simulink model "HILModelFull"  (Simulink 6.6)
settings: Solver=ode4  StartTime=0.0  StopTime=inf  FixedStep=SampleT  RelTol=1e-3
InitFcn:
  | clc
  | Taxi_Var_new
  | failures
  | insInit
  | piccolo_init
values from neighbouring files (symbols this model uses):
  A1 = 0    [Taxi_Var.m]
  Apolar = 0.0899    [Taxi_Var.m]
  CD0 = 0.0219    [Taxi_Var.m]
  chord = S/span    (= 0.384036716878)    [Taxi_Var.m]
  CL0 = 0.1857    [Taxi_Var.m]
  CLa = 4.6206    [Taxi_Var.m]
  CLa_dot = 1.93    [Taxi_Var.m]
  Clb = -0.0043    [Taxi_Var.m]
  ClDa = 0.1695    [Taxi_Var.m]
  CLDe = 0.4032    [Taxi_Var.m]
  CLDf = 0.047    [Taxi_Var.m]
  ClDr = 0.0003    [Taxi_Var.m]
  Clp = -0.4425    [Taxi_Var.m]
  CLq = 8.7465    [Taxi_Var.m]
  Clr = 0.0675    [Taxi_Var.m]
  Cm0 = -0.0902    [Taxi_Var.m]
  Cma = -1.3995    [Taxi_Var.m]
  CmDe = -0.9493    [Taxi_Var.m]
  CmDf = -.021    (= -0.021)    [Taxi_Var.m]
  Cmq = -10.8760    (= -10.876)    [Taxi_Var.m]
  Cnb = 0.0281    [Taxi_Var.m]
  CnDa = -0.0031    [Taxi_Var.m]
  CnDr = -0.0882    [Taxi_Var.m]
  Cnp = -0.0695    [Taxi_Var.m]
  Cnr = -0.1045    [Taxi_Var.m]
  CYb = -0.1999    [Taxi_Var.m]
  CYDr = 0.0192    [Taxi_Var.m]
  damax = 25*deg2rad    (= 0.436332312999)    [Taxi_Var.m]
  damin = -25*deg2rad    (= -0.436332312999)    [Taxi_Var.m]
  datrim = 0*deg2rad    (= 0)    [Taxi_Var.m]
  demax = 15*deg2rad    (= 0.261799387799)    [Taxi_Var.m]
  demin = -15*deg2rad    (= -0.261799387799)    [Taxi_Var.m]
  detrim = -2.4137*deg2rad    (= -0.0421270121554)    [Taxi_Var.m]
  dfland = 30*deg2rad    (= 0.523598775598)    [Taxi_Var.m]
  dfmax = 30*deg2rad    (= 0.523598775598)    [Taxi_Var.m]
  dfmin = 0*deg2rad    (= 0)    [Taxi_Var.m]
  drmax = 25*deg2rad    (= 0.436332312999)    [Taxi_Var.m]
  drmin = -25*deg2rad    (= -0.436332312999)    [Taxi_Var.m]
  drtrim = 0*deg2rad    (= 0)    [Taxi_Var.m]
  dtmax = 1    [Taxi_Var.m]
  dtmin = 0    [Taxi_Var.m]
  dttrim = 0.0725    [Taxi_Var.m]
  Euler_0 = [0; 0; 45]'*pi/180    [Taxi_Var.m]    (also in hilInit.m = [0; 0; 0*pi/180]')
  HIL_K = 3    [hilInit.m]    (also in insInit.m)
  ISA_g = 9.815    [Taxi_Var.m]
  ISA_hmax = 2000    [Taxi_Var.m]
  ISA_lapse = .0065    (= 0.0065)    [Taxi_Var.m]
  ISA_P0 = 101325    [Taxi_Var.m]
  ISA_R = 287    [Taxi_Var.m]
  ISA_rho0 = 1.225    [Taxi_Var.m]
  ISA_T0 = 289    [Taxi_Var.m]
  Ixx = 3.689084    [Taxi_Var.m]
  Iyy = 7.43789    [Taxi_Var.m]
  Izz = 10.22202    [Taxi_Var.m]
  mass = 22.5    [Taxi_Var.m]
  MinThK = 0.075    [Taxi_Var.m]
  Pos_0 = [0; 0; 1000]'    [Taxi_Var.m]    (also in hilInit.m = [500; 750; 350]')
  PQR_0 = [0; 0; 0]'    [Taxi_Var.m]
  span = 2.3368    [Taxi_Var.m]
  TFact = 0.4    [Taxi_Var.m]
  ThK = 2.18    [Taxi_Var.m]
  Vb_0 = [35; 0; 0]'    [Taxi_Var.m]
undefined symbols (not defined in the file or in its folder): clock, Earth, IdxCmdOrbitRadius, IdxCmdOrbitSense, IdxCmdWp1Alt, IdxCmdWp1Lat, IdxCmdWp1Lon, IdxCmdWp2Alt, IdxCmdWp2Lat, IdxCmdWp2Lon, IdxEstimReserved1, IdxEstimWEast, IdxEstimWNorth, IdxGainsAltD, IdxGainsAltI, IdxGainsAltP, IdxGainsPdynD, IdxGainsPdynI, IdxGainsPdynP, IdxGainsPitchD, IdxGainsPitchI, IdxGainsPitchP, IdxGainsRollD, IdxGainsRollI, IdxGainsRollP, IdxGainsSlopeElevatorD, IdxGainsSlopeElevatorP, IdxGainsTrackConv, IdxGainsTrackD, IdxGainsTrackI, IdxGainsTrackP, IdxGainsTurnD, IdxGainsTurnI, IdxGainsTurnP, IdxGainsYawD, IdxGainsYawI, IdxGainsYawP, IdxLimitsAileronMax, IdxLimitsAileronMin, IdxLimitsBankMax, IdxLimitsBankMin, IdxLimitsElevatorMax, IdxLimitsElevatorMin, IdxLimitsFlapMax, IdxLimitsFlapMin, IdxLimitsPdynMax, IdxLimitsPdynMin, IdxLimitsRudderMax, IdxLimitsRudderMin, IdxLimitsThrottleMax, IdxLimitsThrottleMin, IdxSensorsAlt, IdxSensorsLat, IdxSensorsLon, IdxSensorsVDown, IdxSensorsVEast, IdxSensorsVNorth, IdxStatesGlobal, IdxStatesManual, IdxStatesMode ... (+3)
libraries: piccolo_library x60, simulink x33, xpclib x8, aerolibasang x5, aerolibconvert2 x5, aerolibtransform2 x2, aerolibnav x2, aerolibatmos2 x1, dspmtrx3 x1
(part 1 of 4)
CloseFcn:
  | rtwprivate ssgencode ModelCloseRequest AttitudeComplementary
settings Model: Creator=ASL_Lab  LastModifiedBy=UavlabUser
settings DebuggingCC: AlgebraicLoopMsg=error  MultiTaskDSMMsg=warning  MultiTaskCondExecSysMsg=none  StrictBusMsg=None
settings HardwareCC: TargetHWDeviceType=32-bit Generic
settings RTWCC: IncludeERTFirstTime=on

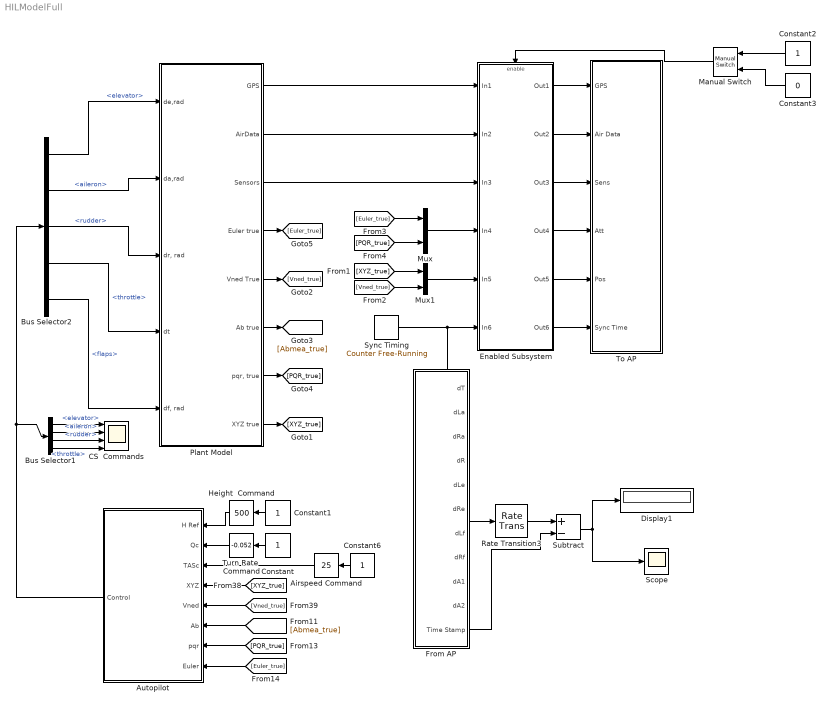
== system HILModelFull ==
  Airspeed Command : simulink/Math Operations/Slider Gain  Orientation=left  SystemSampleTime=-1  low=15  gain=25  high=50
  Autopilot : Subsystem  Orientation=left
  Bus Selector1 : BusSelector  OutputSignals=elevator,aileron,rudder,throttle
  Bus Selector2 : BusSelector  OutputSignals=elevator,aileron,rudder,throttle,flaps
  CS  Commands : Scope  NumInputPorts=4
      settings: TimeRange=44  YMin=0.0142~-2.5e-018~-1e-017~0.665  YMax=0.014425~2e-018~1e-017~0.735  SaveName=ScopeData19
  Constant{,1..2,6} (4 alike) : Constant  Orientation=left
  Constant3 : Constant  Orientation=left  Value=0
  Display1 : Display
  Enabled Subsystem : Subsystem  TreatAsAtomicUnit=on
  From AP : Subsystem
  Height  Command : simulink/Math Operations/Slider Gain  Orientation=left  SystemSampleTime=-1  low=150  gain=500  high=1500
  Manual Switch : simulink/Signal Routing/Manual Switch  Orientation=left  SystemSampleTime=-1  sw=1  action=0  varsize=off
  Mux : Mux  Inputs=2
  Mux1 : Mux  Inputs=2
  Plant Model : Subsystem
  Rate Transition3 : RateTransition  OutPortSampleTime=SampleT
  Scope : Scope
      settings: SaveName=ScopeData2
  Subtract : Sum  Inputs=+-  OutScaling=2^-10
  Sync Timing : simulink/Sources/Counter Free-Running  SystemSampleTime=-1  NumBits=16  tsamp=SampleT*HIL_K
  To AP : Subsystem
  Turn Rate  Command : simulink/Math Operations/Slider Gain  Orientation=left  SystemSampleTime=-1  low=-0.2  gain=-0.052  high=0.2
  wires:
  [XYZ_true] -> Autopilot/4(XYZ)
  [Vned_true] -> Autopilot/5(Vned)
  [Abmea_true] -> Autopilot/6(Ab)
  [PQR_true] -> Autopilot/7(pqr)
  [Euler_true] -> Autopilot/8(Euler)
  Autopilot/1(Control) -> Bus Selector2/1, Bus Selector1/1
  Bus Selector2/1 -> Plant Model/1(de,rad)  "<elevator>"
  Bus Selector2/2 -> Plant Model/2(da,rad)  "<aileron>"
  Bus Selector2/3 -> Plant Model/3("dr, rad")  "<rudder>"
  Bus Selector2/4 -> Plant Model/4(dt)  "<throttle>"
  Bus Selector2/5 -> Plant Model/5("df, rad")  "<flaps>"
  Bus Selector1/1 -> CS  Commands/1  "<elevator>"
  Bus Selector1/2 -> CS  Commands/2  "<aileron>"
  Bus Selector1/3 -> CS  Commands/3  "<rudder>"
  Bus Selector1/4 -> CS  Commands/4  "<throttle>"
  Constant/1 -> Turn Rate  Command/1
  Turn Rate  Command/1 -> Autopilot/2(Qc)
  Constant1/1 -> Height  Command/1
  Height  Command/1 -> Autopilot/1(H Ref)
  Constant6/1 -> Airspeed Command/1
  Airspeed Command/1 -> Autopilot/3(TASc)
  Plant Model/8(XYZ true) -> [XYZ_true]
  Plant Model/5(Vned True) -> [Vned_true]
  Plant Model/6(Ab true) -> [Abmea_true]
  Plant Model/7("pqr, true") -> [PQR_true]
  Plant Model/4(Euler true) -> [Euler_true]
  [PQR_true] -> Mux/2
  [XYZ_true] -> Mux1/1
  [Vned_true] -> Mux1/2
  [Euler_true] -> Mux/1
  Enabled Subsystem/1(Out1) -> To AP/1(GPS)
  Enabled Subsystem/2(Out2) -> To AP/2(Air Data)
  Enabled Subsystem/3(Out3) -> To AP/3(Sens)
  Enabled Subsystem/4(Out4) -> To AP/4(Att)
  Enabled Subsystem/5(Out5) -> To AP/5(Pos)
  Enabled Subsystem/6(Out6) -> To AP/6(Sync Time)
  Plant Model/1(GPS) -> Enabled Subsystem/1(In1)
  Plant Model/2(AirData) -> Enabled Subsystem/2(In2)
  Plant Model/3(Sensors) -> Enabled Subsystem/3(In3)
  Mux/1 -> Enabled Subsystem/4(In4)
  Mux1/1 -> Enabled Subsystem/5(In5)
  Sync Timing/1 -> Enabled Subsystem/6(In6), Rate Transition3/1
  Manual Switch/1 -> Enabled Subsystem/Enable
  Constant2/1 -> Manual Switch/1
  Constant3/1 -> Manual Switch/2
  From AP/11(Time Stamp) -> Subtract/2
  Subtract/1 -> Display1/1, Scope/1
  Rate Transition3/1 -> Subtract/1

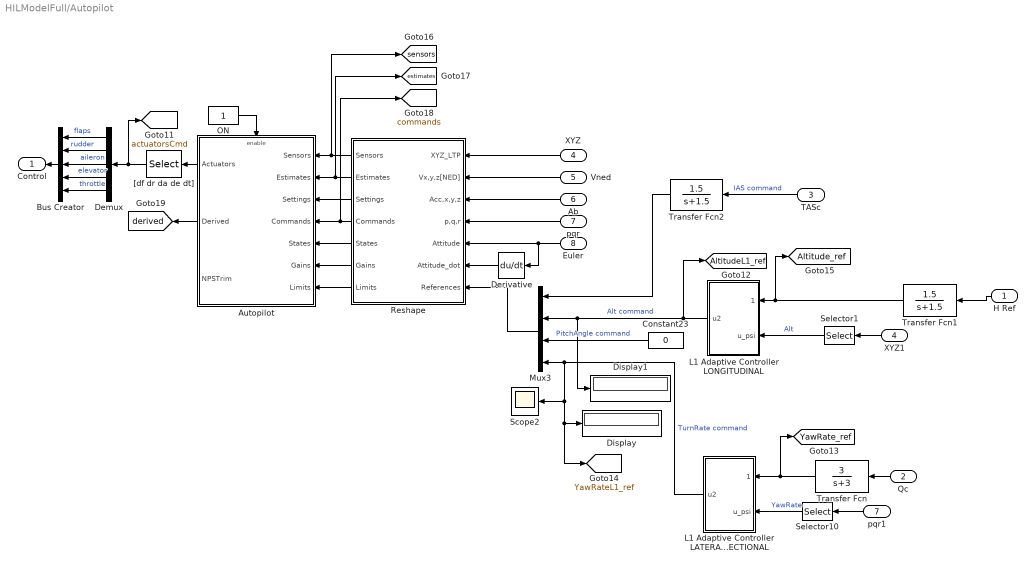
== system HILModelFull/Autopilot ==
  H Ref : Inport  Orientation=left
  Qc : Inport  Orientation=left  Port=2
  TASc : Inport  Orientation=left  Port=3
  XYZ : Inport  Orientation=left  Port=4
  Vned : Inport  Orientation=left  Port=5
  Ab : Inport  Orientation=left  Port=6
  pqr : Inport  Orientation=left  Port=7
  Euler : Inport  Orientation=left  Port=8
  Autopilot : Subsystem  Orientation=left
  Bus Creator : BusCreator  Orientation=left  Inputs=5
  Constant23 : Constant  Orientation=left  Value=0
  Demux : Demux  Orientation=left  Outputs=5
  Derivative : Derivative  Orientation=left
  Display : Display
  Display1 : Display
  L1 Adaptive Controller LATERAL-DIRECTIONAL : Subsystem  Orientation=left  mask{gamma=-2000, m=4, omega=2, Pbound=.1, L1ONOFF=0}
      mask prompts: gamma "L1 gain"; m "state predictor (m)"; omega "low-pass filter (omega)"; Pbound "projection bounds"; L1ONOFF "L1 switch"
  L1 Adaptive Controller LONGITUDINAL : Subsystem  Orientation=left  mask{gamma=-1, m=4, omega=1, Pbound=50, L1ONOFF=0}
      mask prompts: gamma "L1 gain"; m "state predictor (m)"; omega "low-pass filter (omega)"; Pbound "projection bounds"; L1ONOFF "L1 switch"
  Mux3 : Mux  Orientation=left
  ON : Constant
  Reshape : Subsystem  Orientation=left
  Scope2 : Scope
      settings: YMin=-1  YMax=1  SaveName=ScopeData29
  Selector1 : Selector  Orientation=left  IndexOptions=Index vector (dialog)  Indices=3  OutputSizes=1  InputPortWidth=3
  Selector10 : Selector  Orientation=left  IndexOptions=Index vector (dialog)  Indices=3  OutputSizes=1  InputPortWidth=3
  Transfer Fcn : TransferFcn  Orientation=left  Numerator=[3]  Denominator=[1 3]
  Transfer Fcn1 : TransferFcn  Orientation=left  Numerator=[1.5]  Denominator=[1 1.5]
  Transfer Fcn2 : TransferFcn  Orientation=left  Numerator=[1.5]  Denominator=[1 1.5]
  XYZ1 : InportShadow  Orientation=left  Port=4  LatchByCopyingInsideSignal=off
  "[df dr da de dt]" : Selector  Orientation=left  IndexOptions=Index vector (dialog)  Indices=[10 6 2 4 8]  OutputSizes=[(-2)]  InputPortWidth=12
  pqr1 : InportShadow  Orientation=left  Port=7  LatchByCopyingInsideSignal=off
  Control : Outport  Orientation=left
  tag scope: AltitudeL1_ref=global, Altitude_ref=global, YawRateL1_ref=global, YawRate_ref=global, actuatorsCmd=global, commands=global, derived=global, estimates=global, sensors=global
  wires:
  XYZ/1 -> Reshape/1(XYZ_LTP)
  Vned/1 -> Reshape/2(Vx,y,z[NED])
  Ab/1 -> Reshape/3(Acc,x,y,z)
  pqr/1 -> Reshape/4(p,q,r)
  Reshape/1(Sensors) -> Autopilot/1(Sensors), [sensors]
  Reshape/2(Estimates) -> Autopilot/2(Estimates), [estimates]
  Reshape/3(Settings) -> Autopilot/3(Settings)
  Reshape/4(Commands) -> Autopilot/4(Commands), [commands]
  Reshape/5(States) -> Autopilot/5(States)
  Reshape/6(Gains) -> Autopilot/6(Gains)
  Reshape/7(Limits) -> Autopilot/7(Limits)
  ON/1 -> Autopilot/Enable
  Autopilot/1(Actuators) -> "[df dr da de dt]"/1
  "[df dr da de dt]"/1 -> Demux/1, [actuatorsCmd]
  Euler/1 -> Reshape/5(Attitude), Derivative/1
  Autopilot/2(Derived) -> [derived]
  TASc/1 -> Transfer Fcn2/1  "IAS command"
  L1 Adaptive Controller LONGITUDINAL/1(u2) -> [AltitudeL1_ref], Mux3/2, Display1/1  "Alt command"
  Constant23/1 -> Mux3/3  "PitchAngle command"
  L1 Adaptive Controller LATERAL-DIRECTIONAL/1(u2) -> Mux3/4, Display/1, [YawRateL1_ref], Scope2/1  "TurnRate command"
  Mux3/1 -> Reshape/7(References)
  Qc/1 -> Transfer Fcn/1
  pqr1/1 -> Selector10/1
  Selector10/1 -> L1 Adaptive Controller LATERAL-DIRECTIONAL/2(u_psi)  "YawRate"
  H Ref/1 -> Transfer Fcn1/1
  XYZ1/1 -> Selector1/1
  Selector1/1 -> L1 Adaptive Controller LONGITUDINAL/2(u_psi)  "Alt"
  Demux/1 -> Bus Creator/1  "flaps"
  Demux/2 -> Bus Creator/2  "rudder"
  Demux/3 -> Bus Creator/3  "aileron"
  Demux/4 -> Bus Creator/4  "elevator"
  Demux/5 -> Bus Creator/5  "throttle"
  Bus Creator/1 -> Control/1
  Transfer Fcn/1 -> L1 Adaptive Controller LATERAL-DIRECTIONAL/1(u_psi_c), [YawRate_ref]
  Transfer Fcn1/1 -> L1 Adaptive Controller LONGITUDINAL/1(u_psi_c), [Altitude_ref]
  Transfer Fcn2/1 -> Mux3/1
  Derivative/1 -> Reshape/6(Attitude_dot)

== system HILModelFull/Enabled Subsystem ==
  In1 : Inport
  In2 : Inport  Port=2
  In3 : Inport  Port=3
  In4 : Inport  Port=4
  In5 : Inport  Port=5
  In6 : Inport  Port=6
  Enable : EnablePort
  Out1 : Outport
  Out2 : Outport  Port=2
  Out3 : Outport  Port=3
  Out4 : Outport  Port=4
  Out5 : Outport  Port=5
  Out6 : Outport  Port=6
  wires:
  In1/1 -> Out1/1
  In2/1 -> Out2/1
  In3/1 -> Out3/1
  In4/1 -> Out4/1
  In5/1 -> Out5/1
  In6/1 -> Out6/1

== system HILModelFull/From AP ==
  Bus Creator : BusCreator  Inputs=11
  Bus Selector : BusSelector  OutputSignals=dt,dla,dra,dr,dle,dre,dlf,drf,da1,da2,timeStamp
  Data Type Conversion{1..11} (11 alike) : DataTypeConversion  OutDataTypeMode=double
  Receive : xpclib/UDP/Receive  ipAddress=0.0.0.0  ipPort=5678  width=22  sampletime=SampleT
  Terminator : Terminator
  Unpack1 : xpclib/UDP/Unpack  dimensions={1,1,1,1,1,1,1,1,1,1,1}  datatypes={'uint16','uint16','uint16','uint16', 'uint16', 'uint16','uint16', 'uint16','uint16', 'uint16','uint16'}  byteAlign=1
  dT : Outport
  dLa : Outport  Port=2
  dRa : Outport  Port=3
  dR : Outport  Port=4
  dLe : Outport  Port=5
  dRe : Outport  Port=6
  dLf : Outport  Port=7
  dRf : Outport  Port=8
  dA1 : Outport  Port=9
  dA2 : Outport  Port=10
  Time Stamp : Outport  Port=11
  wires:
  Receive/1 -> Unpack1/1
  Receive/2 -> Terminator/1
  Bus Creator/1 -> Bus Selector/1
  Data Type Conversion1/1 -> dT/1
  Data Type Conversion2/1 -> dLa/1
  Data Type Conversion3/1 -> dRa/1
  Data Type Conversion4/1 -> dR/1
  Data Type Conversion5/1 -> dLe/1
  Data Type Conversion6/1 -> dRe/1
  Data Type Conversion7/1 -> dLf/1
  Data Type Conversion8/1 -> dRf/1
  Data Type Conversion9/1 -> dA1/1
  Data Type Conversion10/1 -> dA2/1
  Unpack1/1 -> Bus Creator/1  "dt"
  Unpack1/3 -> Bus Creator/3  "dra"
  Unpack1/5 -> Bus Creator/5  "dle"
  Unpack1/7 -> Bus Creator/7  "dlf"
  Unpack1/9 -> Bus Creator/9  "da1"
  Unpack1/11 -> Bus Creator/11  "timeStamp"
  Data Type Conversion11/1 -> Time Stamp/1
  Bus Selector/1 -> Data Type Conversion1/1  "<dt>"
  Bus Selector/2 -> Data Type Conversion2/1  "<dla>"
  Bus Selector/3 -> Data Type Conversion3/1  "<dra>"
  Bus Selector/4 -> Data Type Conversion4/1  "<dr>"
  Bus Selector/5 -> Data Type Conversion5/1  "<dle>"
  Bus Selector/6 -> Data Type Conversion6/1  "<dre>"
  Bus Selector/7 -> Data Type Conversion7/1  "<dlf>"
  Bus Selector/8 -> Data Type Conversion8/1  "<drf>"
  Bus Selector/9 -> Data Type Conversion9/1  "<da1>"
  Bus Selector/10 -> Data Type Conversion10/1  "<da2>"
  Bus Selector/11 -> Data Type Conversion11/1  "<timeStamp>"
  Unpack1/2 -> Bus Creator/2  "dla"
  Unpack1/4 -> Bus Creator/4  "dr"
  Unpack1/6 -> Bus Creator/6  "dre"
  Unpack1/8 -> Bus Creator/8  "drf"
  Unpack1/10 -> Bus Creator/10  "da2"

== system HILModelFull/Plant Model ==
  de,rad : Inport
  da,rad : Inport  Port=2
  "dr, rad" : Inport  Port=3
  dt : Inport  Port=4
  "df, rad" : Inport  Port=5
  Angle Conversion{,1..3} (4 alike) : aerolibconvert2/Angle Conversion  SystemSampleTime=-1  IU=rad  OU=deg
  Constant : Constant  Value=18  SampleTime=SampleT
  Constant1 : Constant  SampleTime=SampleT
  Constant2 : Constant  Value=7  SampleTime=SampleT
  Constant3 : Constant  SampleTime=SampleT
  Generic Sensor : Subsystem  AncestorBlock=aerolibnav/Three-axis Gyroscope  mask(Sensor){dtype_g=off, w_g=190, z_g=0.707, g_sf_cc=[2.076 0 0; 0 .0349 0; 0 0 28.237], g_bias=[-67.805 -141.8 -6376.1], g_sen=[0 0 0], g_rand=on, g_seeds=[23093 23094 23095], g_pow=[0.008 0.008 0.008], g_sat=[-inf  -inf  -inf  inf inf inf], g_Ts=SampleT}
      mask prompts: dtype_g "Second-order dynamics"; w_g "Natural frequency (rad/sec):"; z_g "Damping ratio:"; g_sf_cc "Scale factors and cross-coupling:"; g_bias "Measurement bias:"; g_sen "G-sensitive bias:"; g_rand "Noise on"; g_seeds "Noise seeds:"; g_pow "Noise power:"; g_sat "Lower and upper output limits:"; g_Ts "Update rate (sec):"
      mask help: Implement a reading to Sensor out
      mask TabNameString: Main,Main,Main,Main,Main,Main,Noise,Noise,Noise,Noise,Main
  Mux : Mux  Inputs=15
  Mux1 : Mux  Inputs=3
  Plant : Subsystem
  Subsystem : Subsystem
  GPS : Outport
  AirData : Outport  Port=2
  Sensors : Outport  Port=3
  Euler true : Outport  Port=4
  Vned True : Outport  Port=5
  Ab true : Outport  Port=6
  "pqr, true" : Outport  Port=7
  XYZ true : Outport  Port=8
  wires:
  de,rad/1 -> Angle Conversion/1
  da,rad/1 -> Angle Conversion1/1
  "dr, rad"/1 -> Angle Conversion2/1
  dt/1 -> Plant/4(dt)
  "df, rad"/1 -> Angle Conversion3/1
  Angle Conversion/1 -> Plant/1(de)
  Angle Conversion1/1 -> Plant/2(da)
  Angle Conversion2/1 -> Plant/3(dr)
  Angle Conversion3/1 -> Plant/5(df)
  Mux/1 -> GPS/1
  Plant/1(GPS Year) -> Mux/1
  Plant/2(GPS Month) -> Mux/2
  Plant/3(GPS Day) -> Mux/3
  Plant/4(GPS Hr) -> Mux/4
  Plant/5(GPS Min) -> Mux/5
  Plant/6(GPS Sec) -> Mux/6
  Plant/7(GPS Lat (deg)) -> Mux/7
  Plant/8(GPS Long (deg)) -> Mux/8
  Plant/9(GPS H (m)) -> Mux/9
  Plant/10(COG (deg)) -> Mux/10
  Plant/11(SOG(m/s)) -> Mux/11
  Plant/12(Dynamic) -> Mux1/1
  Plant/13(Static) -> Mux1/2
  Plant/14(OAT) -> Mux1/3
  Mux1/1 -> Generic Sensor/1(Sens)
  Subsystem/1(Sens) -> Sensors/1
  Plant/15(PQR) -> Subsystem/1(PQR), "pqr, true"/1
  Plant/16(Ab meas) -> Subsystem/2(Ab), Ab true/1
  Plant/17("Mag, nT") -> Subsystem/3(Mag)
  Constant/1 -> Mux/12
  Constant1/1 -> Mux/13
  Constant2/1 -> Mux/14
  Constant3/1 -> Mux/15
  Generic Sensor/1(Meas) -> AirData/1
  Plant/18(Euler) -> Euler true/1
  Plant/20(Vned) -> Vned True/1
  Plant/22(XYZ) -> XYZ true/1

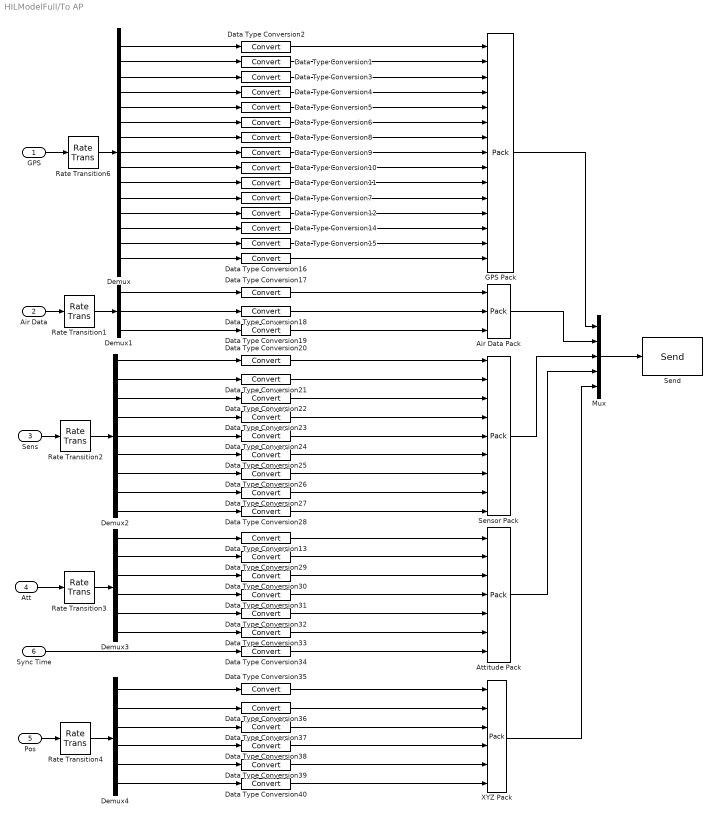
== system HILModelFull/To AP ==
  GPS : Inport
  Air Data : Inport  Port=2
  Sens : Inport  Port=3
  Att : Inport  Port=4
  Pos : Inport  Port=5
  Sync Time : Inport  Port=6
  Air Data Pack : xpclib/UDP/Pack  datatypes={'single', 'single', 'int16'}  byteAlign=1
  Attitude Pack : xpclib/UDP/Pack  datatypes={'single','single','single','single','single','single','uint16'}  byteAlign=1
  Data Type Conversion{1..6,14..16} (9 alike) : DataTypeConversion  OutDataTypeMode=uint8
  Data Type Conversion{8..10,13,17..18,29..33,35..40} (17 alike) : DataTypeConversion  OutDataTypeMode=single
  Data Type Conversion{7,11..12,20..28,34} (13 alike) : DataTypeConversion  OutDataTypeMode=uint16
  Data Type Conversion19 : DataTypeConversion  OutDataTypeMode=int16
  Demux : Demux  Outputs=15
  Demux1 : Demux  Outputs=3
  Demux2 : Demux  Outputs=9
  Demux3 : Demux  Outputs=6
  Demux4 : Demux  Outputs=6
  GPS Pack : xpclib/UDP/Pack  datatypes={'uint8','uint8','uint8','uint8','uint8','uint8', 'single', 'single', 'single', 'uint16', 'uint16', 'uint16', 'uint8', 'uint8', 'uint8'}  byteAlign=1
  Mux : Mux  Inputs=5
  Rate Transition{1..4,6} (5 alike) : RateTransition  OutPortSampleTime=SampleT*HIL_K
  Send : xpclib/UDP/Send  ipAddress=255.255.255.255  ipPort=5679  localPort=5678  sampletime=SampleT*HIL_K
  Sensor Pack : xpclib/UDP/Pack  datatypes={'uint16', 'uint16', 'uint16', 'uint16', 'uint16', 'uint16', 'uint16', 'uint16', 'uint16'}  byteAlign=1
  XYZ Pack : xpclib/UDP/Pack  datatypes={'single','single','single','single','single','single'}  byteAlign=1
  wires:
  Demux/1 -> Data Type Conversion2/1
  Demux/2 -> Data Type Conversion1/1
  Demux/3 -> Data Type Conversion3/1
  Demux/4 -> Data Type Conversion4/1
  Demux/5 -> Data Type Conversion5/1
  Demux/6 -> Data Type Conversion6/1
  Demux/7 -> Data Type Conversion8/1
  Demux/8 -> Data Type Conversion9/1
  Demux/9 -> Data Type Conversion10/1
  Demux/10 -> Data Type Conversion11/1
  Demux/11 -> Data Type Conversion7/1
  Demux/12 -> Data Type Conversion12/1
  Demux/13 -> Data Type Conversion14/1
  Demux/14 -> Data Type Conversion15/1
  Demux/15 -> Data Type Conversion16/1
  Demux1/1 -> Data Type Conversion17/1
  Demux1/2 -> Data Type Conversion18/1
  Demux1/3 -> Data Type Conversion19/1
  Demux2/1 -> Data Type Conversion20/1
  Demux2/2 -> Data Type Conversion21/1
  Demux2/3 -> Data Type Conversion22/1
  Demux2/4 -> Data Type Conversion23/1
  Demux2/5 -> Data Type Conversion24/1
  Demux2/6 -> Data Type Conversion25/1
  Demux2/7 -> Data Type Conversion26/1
  Demux2/8 -> Data Type Conversion27/1
  Demux2/9 -> Data Type Conversion28/1
  Mux/1 -> Send/1
  GPS Pack/1 -> Mux/1
  Air Data Pack/1 -> Mux/2
  Sensor Pack/1 -> Mux/3
  GPS/1 -> Rate Transition6/1
  Air Data/1 -> Rate Transition1/1
  Sens/1 -> Rate Transition2/1
  Rate Transition6/1 -> Demux/1
  Rate Transition1/1 -> Demux1/1
  Rate Transition2/1 -> Demux2/1
  Att/1 -> Rate Transition3/1
  Pos/1 -> Rate Transition4/1
  Rate Transition3/1 -> Demux3/1
  Demux3/1 -> Data Type Conversion13/1
  Demux3/2 -> Data Type Conversion29/1
  Demux3/3 -> Data Type Conversion30/1
  Demux3/4 -> Data Type Conversion31/1
  Demux3/5 -> Data Type Conversion32/1
  Demux3/6 -> Data Type Conversion33/1
  Demux4/1 -> Data Type Conversion35/1
  Demux4/2 -> Data Type Conversion36/1
  Demux4/3 -> Data Type Conversion37/1
  Demux4/4 -> Data Type Conversion38/1
  Demux4/5 -> Data Type Conversion39/1
  Demux4/6 -> Data Type Conversion40/1
  Rate Transition4/1 -> Demux4/1
  Attitude Pack/1 -> Mux/4
  XYZ Pack/1 -> Mux/5
  Sync Time/1 -> Data Type Conversion34/1
  Data Type Conversion2/1 -> GPS Pack/1
  Data Type Conversion1/1 -> GPS Pack/2
  Data Type Conversion3/1 -> GPS Pack/3
  Data Type Conversion4/1 -> GPS Pack/4
  Data Type Conversion5/1 -> GPS Pack/5
  Data Type Conversion6/1 -> GPS Pack/6
  Data Type Conversion8/1 -> GPS Pack/7
  Data Type Conversion9/1 -> GPS Pack/8
  Data Type Conversion10/1 -> GPS Pack/9
  Data Type Conversion11/1 -> GPS Pack/10
  Data Type Conversion7/1 -> GPS Pack/11
  Data Type Conversion12/1 -> GPS Pack/12
  Data Type Conversion14/1 -> GPS Pack/13
  Data Type Conversion15/1 -> GPS Pack/14
  Data Type Conversion16/1 -> GPS Pack/15
  Data Type Conversion17/1 -> Air Data Pack/1
  Data Type Conversion18/1 -> Air Data Pack/2
  Data Type Conversion19/1 -> Air Data Pack/3
  Data Type Conversion20/1 -> Sensor Pack/1
  Data Type Conversion21/1 -> Sensor Pack/2
  Data Type Conversion22/1 -> Sensor Pack/3
  Data Type Conversion23/1 -> Sensor Pack/4
  Data Type Conversion24/1 -> Sensor Pack/5
  Data Type Conversion25/1 -> Sensor Pack/6
  Data Type Conversion26/1 -> Sensor Pack/7
  Data Type Conversion27/1 -> Sensor Pack/8
  Data Type Conversion28/1 -> Sensor Pack/9
  Data Type Conversion13/1 -> Attitude Pack/1
  Data Type Conversion29/1 -> Attitude Pack/2
  Data Type Conversion30/1 -> Attitude Pack/3
  Data Type Conversion31/1 -> Attitude Pack/4
  Data Type Conversion32/1 -> Attitude Pack/5
  Data Type Conversion33/1 -> Attitude Pack/6
  Data Type Conversion34/1 -> Attitude Pack/7
  Data Type Conversion35/1 -> XYZ Pack/1
  Data Type Conversion36/1 -> XYZ Pack/2
  Data Type Conversion37/1 -> XYZ Pack/3
  Data Type Conversion38/1 -> XYZ Pack/4
  Data Type Conversion39/1 -> XYZ Pack/5
  Data Type Conversion40/1 -> XYZ Pack/6

== system HILModelFull/Autopilot/Autopilot ==
  Sensors : Inport  PortDimensions=SizeSensors
  Estimates : Inport  Port=2  PortDimensions=SizeEstim
  Settings : Inport  Port=3  PortDimensions=SizeSet
  Commands : Inport  Port=4  PortDimensions=SizeCmd
  States : Inport  Port=5  PortDimensions=SizeStates
  Gains : Inport  Port=6  PortDimensions=SizeGains
  Limits : Inport  Port=7  PortDimensions=SizeLimits
  Autopilot Enable : EnablePort  StatesWhenEnabling=reset
  Air System Vector Inputs : piccolo_library/Flight Mechanics/Air System Vector Inputs  SystemSampleTime=-1  tsamp=APtsamp
  Altitude Control Vector Inputs : Subsystem  AncestorBlock=piccolo_library/Controllers/Longitudinal/Altitude Control Vector Inputs
  Demux{,1..6} (7 alike) : Demux  Outputs=7
  Flap Control Vector Inputs : Subsystem
  Gain : Gain  SaturateOnIntegerOverflow=on
  Gain1 : Gain  SaturateOnIntegerOverflow=on
  Guidance & Navigation Vector Input : Subsystem  AncestorBlock=piccolo_library/Controllers/Guidance/Guidance & Navigation Vector Input
  Mux : Mux  Inputs=12
  Mux1 : Mux  Inputs=5
  Mux2 : Mux  Inputs=7
  Pitch Control  Vector Inputs : Subsystem  AncestorBlock="piccolo_library/Controllers/Longitudinal/Pitch Control  Vector Inputs"
  Reserved Outputs : Constant  Value=0
  Roll Control Vector Inputs : Subsystem  AncestorBlock=piccolo_library/Controllers/Lateral/Roll Control Vector Inputs
  Yaw Control Vector Inputs : Subsystem  AncestorBlock=piccolo_library/Controllers/Lateral/Yaw Control Vector Inputs
  Actuators : Outport  OutDataType=fixdt(1,16,0)  OutScaling=[]
  Derived : Outport  Port=2  OutDataType=fixdt(1,16,0)  OutScaling=[]
  NPSTrim : Outport  Port=3  OutDataType=fixdt(1,16,0)  OutScaling=[]  InitialOutput=0
  wires:
  Mux/1 -> Gain/1, NPSTrim/1
  Mux1/1 -> Roll Control Vector Inputs/8(Derived), Altitude Control Vector Inputs/8(Derived), Pitch Control  Vector Inputs/8(Derived), Guidance & Navigation Vector Input/8(Derived), Yaw Control Vector Inputs/8(Derived), Air System Vector Inputs/8, Flap Control Vector Inputs/8(Derived), Gain1/1
  Roll Control Vector Inputs/1(Actuator) -> Mux/2
  Pitch Control  Vector Inputs/1(Actuator) -> Mux/4
  Altitude Control Vector Inputs/1(Actuator) -> Mux/8
  Sensors/1 -> Mux2/1
  Estimates/1 -> Mux2/2
  Settings/1 -> Mux2/3
  Commands/1 -> Mux2/4
  States/1 -> Mux2/5
  Gains/1 -> Mux2/6
  Limits/1 -> Mux2/7
  Demux/1 -> Altitude Control Vector Inputs/1(Sensors)
  Demux/2 -> Altitude Control Vector Inputs/2(Estimates)
  Demux/3 -> Altitude Control Vector Inputs/3(Settings)
  Demux/4 -> Altitude Control Vector Inputs/4(Commands)
  Demux/5 -> Altitude Control Vector Inputs/5(States)
  Demux/6 -> Altitude Control Vector Inputs/6(Gains)
  Demux/7 -> Altitude Control Vector Inputs/7(Limits)
  Demux1/1 -> Roll Control Vector Inputs/1(Sensors)
  Demux1/2 -> Roll Control Vector Inputs/2(Estimates)
  Demux1/3 -> Roll Control Vector Inputs/3(Settings)
  Demux1/4 -> Roll Control Vector Inputs/4(Commands)
  Demux1/5 -> Roll Control Vector Inputs/5(States)
  Demux1/6 -> Roll Control Vector Inputs/6(Gains)
  Demux1/7 -> Roll Control Vector Inputs/7(Limits)
  Demux2/1 -> Pitch Control  Vector Inputs/1(Sensors)
  Demux2/2 -> Pitch Control  Vector Inputs/2(Estimates)
  Demux2/3 -> Pitch Control  Vector Inputs/3(Settings)
  Demux2/4 -> Pitch Control  Vector Inputs/4(Commands)
  Demux2/5 -> Pitch Control  Vector Inputs/5(States)
  Demux2/6 -> Pitch Control  Vector Inputs/6(Gains)
  Demux2/7 -> Pitch Control  Vector Inputs/7(Limits)
  Demux3/1 -> Guidance & Navigation Vector Input/1(Sensors)
  Demux3/2 -> Guidance & Navigation Vector Input/2(Estimates)
  Demux3/3 -> Guidance & Navigation Vector Input/3(Settings)
  Demux3/4 -> Guidance & Navigation Vector Input/4(Commands)
  Demux3/5 -> Guidance & Navigation Vector Input/5(States)
  Demux3/6 -> Guidance & Navigation Vector Input/6(Gains)
  Demux3/7 -> Guidance & Navigation Vector Input/7(Limits)
  Demux4/1 -> Yaw Control Vector Inputs/1(Sensors)
  Demux4/2 -> Yaw Control Vector Inputs/2(Estimates)
  Demux4/3 -> Yaw Control Vector Inputs/3(Settings)
  Demux4/4 -> Yaw Control Vector Inputs/4(Commands)
  Demux4/5 -> Yaw Control Vector Inputs/5(States)
  Demux4/6 -> Yaw Control Vector Inputs/6(Gains)
  Demux4/7 -> Yaw Control Vector Inputs/7(Limits)
  Demux5/1 -> Air System Vector Inputs/1
  Demux5/2 -> Air System Vector Inputs/2
  Demux5/3 -> Air System Vector Inputs/3
  Demux5/4 -> Air System Vector Inputs/4
  Demux5/5 -> Air System Vector Inputs/5
  Demux5/6 -> Air System Vector Inputs/6
  Demux5/7 -> Air System Vector Inputs/7
  Mux2/1 -> Demux1/1, Demux/1, Demux2/1, Demux3/1, Demux4/1, Demux5/1, Demux6/1
  Reserved Outputs/1 -> Mux/11, Mux/9, Mux/7, Mux/1, Mux/3, Mux/5, Mux/12
  Yaw Control Vector Inputs/1(Actuator) -> Mux/6
  Flap Control Vector Inputs/1(Actuator) -> Mux/10
  Demux6/1 -> Flap Control Vector Inputs/1(Sensors)
  Demux6/2 -> Flap Control Vector Inputs/2(Estimates)
  Demux6/3 -> Flap Control Vector Inputs/3(Settings)
  Demux6/4 -> Flap Control Vector Inputs/4(Commands)
  Demux6/5 -> Flap Control Vector Inputs/5(States)
  Demux6/6 -> Flap Control Vector Inputs/6(Gains)
  Demux6/7 -> Flap Control Vector Inputs/7(Limits)
  Air System Vector Inputs/1 -> Mux1/1
  Roll Control Vector Inputs/2(Param) -> Mux1/2
  Pitch Control  Vector Inputs/2(Param) -> Mux1/3
  Guidance & Navigation Vector Input/1(Param) -> Mux1/4
  Altitude Control Vector Inputs/2(Param) -> Mux1/5
  Gain/1 -> Actuators/1
  Gain1/1 -> Derived/1

== system HILModelFull/Autopilot/L1 Adaptive Controller LATERAL-DIRECTIONAL ==
  u_psi_c : Inport
  u_psi : Inport  Port=2
  Display : Display
  Mux2 : Mux  Inputs=2
  PF Yaw Channel L1 Augmentation : Subsystem  Orientation=left
  Scope1 : Scope  NumInputPorts=2
      settings: YMin=0.0999875~-4.5e-005  YMax=0.100045~1.25e-005  SaveName=ScopeData28
  Sum1 : Sum  Inputs=-+|
  Sum2 : Sum  Inputs=-+|
  u2 : Outport
  wires:
  u_psi/1 -> PF Yaw Channel L1 Augmentation/1(u_psi), Mux2/2, Sum2/1
  PF Yaw Channel L1 Augmentation/1(C_sighat_2) -> Sum1/1, Display/1  "L1 augmentation"
  u_psi_c/1 -> Sum1/2, Mux2/1, Sum2/2
  Sum1/1 -> u2/1, PF Yaw Channel L1 Augmentation/2(u2)
  Mux2/1 -> Scope1/1
  Sum2/1 -> Scope1/2

== system HILModelFull/Autopilot/L1 Adaptive Controller LONGITUDINAL ==
  u_psi_c : Inport
  u_psi : Inport  Port=2
  Display : Display
  Mux2 : Mux  Inputs=2
  PF Yaw Channel L1 Augmentation : Subsystem  Orientation=left
  Scope1 : Scope  NumInputPorts=2
      settings: YMin=0.0999875~-4.5e-005  YMax=0.100045~1.25e-005  SaveName=ScopeData28
  Sum1 : Sum  Inputs=-+|
  Sum2 : Sum  Inputs=-+|
  u2 : Outport
  wires:
  Sum2/1 -> Scope1/2
  Mux2/1 -> Scope1/1
  Sum1/1 -> PF Yaw Channel L1 Augmentation/2(u2), u2/1
  u_psi_c/1 -> Sum2/2, Mux2/1, Sum1/2
  PF Yaw Channel L1 Augmentation/1(C_sighat_2) -> Display/1, Sum1/1  "L1 augmentation"
  u_psi/1 -> Sum2/1, Mux2/2, PF Yaw Channel L1 Augmentation/1(u_psi)

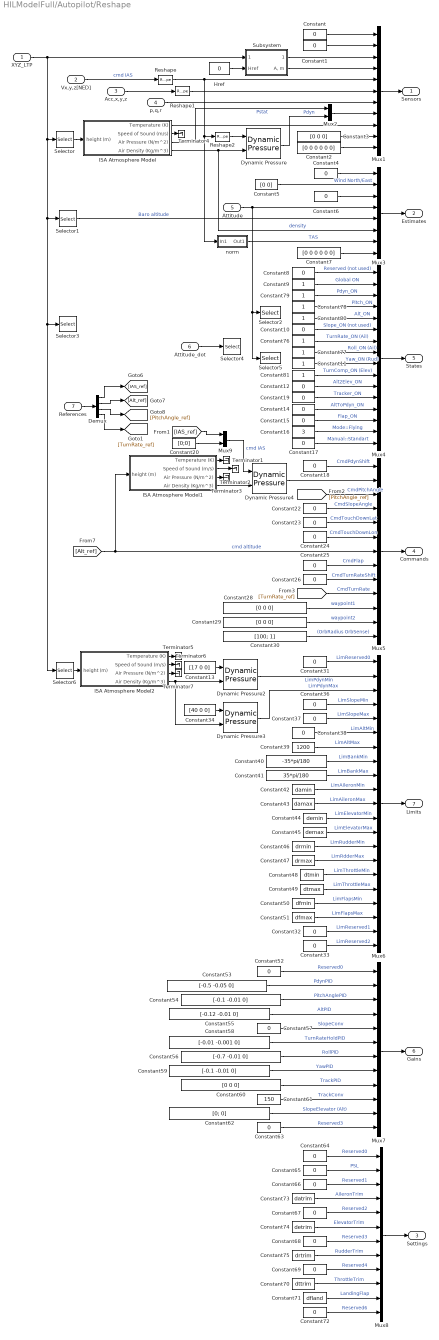
== system HILModelFull/Autopilot/Reshape ==
  XYZ_LTP : Inport  OutDataType=fixdt(1,16,0)  OutScaling=[]
  Vx,y,z[NED] : Inport  Port=2  OutDataType=fixdt(1,16,0)  OutScaling=[]
  Acc,x,y,z : Inport  Port=3  OutDataType=fixdt(1,16,0)  OutScaling=[]
  p,q,r : Inport  Port=4  OutDataType=fixdt(1,16,0)  OutScaling=[]
  Attitude : Inport  Port=5  OutDataType=fixdt(1,16,0)  OutScaling=[]
  Attitude_dot : Inport  Port=6  OutDataType=fixdt(1,16,0)  OutScaling=[]
  References : Inport  Port=7  OutDataType=fixdt(1,16,0)  OutScaling=[]
  Constant{,1,4,6,8,10,12,14..15,17..19,22..26,31..33,36..38,52,57,63..69,72} (33 alike) : Constant  Value=0
  Constant{9,11,76..81} (8 alike) : Constant
  Constant13 : Constant  Value=[17 0 0]
  Constant16 : Constant  Value=3
  Constant2 : Constant  Value=[0 0 0 0 0 0]
  Constant20 : Constant  Value=[0;0]
  Constant{3,28..29,60} (4 alike) : Constant  Value=[0 0 0]
  Constant30 : Constant  Value=[100; 1]
  Constant34 : Constant  Value=[40 0 0]
  Constant39 : Constant  Value=1200
  Constant40 : Constant  Value=-35*pi/180
  Constant41 : Constant  Value=35*pi/180
  Constant42 : Constant  Value=damin
  Constant43 : Constant  Value=damax
  Constant44 : Constant  Value=demin
  Constant45 : Constant  Value=demax
  Constant46 : Constant  Value=drmin
  Constant47 : Constant  Value=drmax
  Constant48 : Constant  Value=dtmin
  Constant49 : Constant  Value=dtmax
  Constant5 : Constant  Value=[0 0]
  Constant50 : Constant  Value=dfmin
  Constant51 : Constant  Value=dfmax
  Constant53 : Constant  Value=[-0.5 -0.05 0]
  Constant54 : Constant  Value=[-0.1 -0.01 0]
  Constant55 : Constant  Value=[-0.12 -0.01 0]
  Constant56 : Constant  Value=[-0.7 -0.01 0]
  Constant58 : Constant  Value=[-0.01 -0.001 0]
  Constant59 : Constant  Value=[-0.1 -0.01 0]
  Constant61 : Constant  Value=150
  Constant62 : Constant  Value=[0; 0]
  Constant7 : Constant  Value=[0 0 0 0 0 0]
  Constant70 : Constant  Value=dttrim
  Constant71 : Constant  Value=dfland
  Constant73 : Constant  Value=datrim
  Constant74 : Constant  Value=detrim
  Constant75 : Constant  Value=drtrim
  Demux : Demux
  Dynamic Pressure{,2..4} (4 alike) : aerolibasang/Dynamic Pressure  SystemSampleTime=-1
  Href : Constant  Value=0
  ISA Atmosphere Model : Subsystem  mask(International Standart Atmosphere){L=ISA_lapse, h_lim=ISA_hmax, R=ISA_R, g=ISA_g, rh0=ISA_rho0, P0=ISA_P0, T0=ISA_T0}
      mask prompts: L "Lapse rate"; h_lim "Upper altitude limit, (m)"; R "Universal gas constant R"; g "Garvity constant, (m/c^2)"; rh0 "Sea level density, (kg/m^3)"; P0 "Sea level pressure, (N/m^2)"; T0 "Sea level temperature, (K)"
  ISA Atmosphere Model1 : Subsystem  mask(International Standart Atmosphere){L=ISA_lapse, h_lim=ISA_hmax, R=ISA_R, g=ISA_g, rh0=ISA_rho0, P0=ISA_P0, T0=ISA_T0}
      mask prompts: L "Lapse rate"; h_lim "Upper altitude limit, (m)"; R "Universal gas constant R"; g "Garvity constant, (m/c^2)"; rh0 "Sea level density, (kg/m^3)"; P0 "Sea level pressure, (N/m^2)"; T0 "Sea level temperature, (K)"
  ISA Atmosphere Model2 : Subsystem  mask(International Standart Atmosphere){L=ISA_lapse, h_lim=ISA_hmax, R=ISA_R, g=ISA_g, rh0=ISA_rho0, P0=ISA_P0, T0=ISA_T0}
      mask prompts: L "Lapse rate"; h_lim "Upper altitude limit, (m)"; R "Universal gas constant R"; g "Garvity constant, (m/c^2)"; rh0 "Sea level density, (kg/m^3)"; P0 "Sea level pressure, (N/m^2)"; T0 "Sea level temperature, (K)"
  Mux1 : Mux  Inputs=11
  Mux2 : Mux  Inputs=2
  Mux3 : Mux  Inputs=8
  Mux4 : Mux  Inputs=16
  Mux5 : Mux  Inputs=13
  Mux6 : Mux  Inputs=21
  Mux7 : Mux  Inputs=12
  Mux8 : Mux  Inputs=12
  Mux9 : Mux  Inputs=2
  Reshape : Reshape
  Reshape1 : Reshape
  Reshape2 : Reshape
  Selector{,1,3..4,6} (5 alike) : Selector  IndexOptions=Index vector (dialog)  Indices=3  OutputSizes=[(-2)]  InputPortWidth=3
  Selector2 : Selector  IndexOptions=Index vector (dialog)  Indices=2  OutputSizes=[(-2)]  InputPortWidth=3
  Selector5 : Selector  IndexOptions=Index vector (dialog)  Indices=[1 3]  OutputSizes=[(-2)]  InputPortWidth=3
  Subsystem : Subsystem
  Terminator{1..7} (7 alike) : Terminator
  norm : Subsystem
  Sensors : Outport  OutDataType=fixdt(1,16,0)  OutScaling=[]
  Estimates : Outport  Port=2  OutDataType=fixdt(1,16,0)  OutScaling=[]
  Settings : Outport  Port=3  OutDataType=fixdt(1,16,0)  OutScaling=[]
  Commands : Outport  Port=4  OutDataType=fixdt(1,16,0)  OutScaling=[]
  States : Outport  Port=5  OutDataType=fixdt(1,16,0)  OutScaling=[]
  Gains : Outport  Port=6  OutDataType=fixdt(1,16,0)  OutScaling=[]
  Limits : Outport  Port=7  OutDataType=fixdt(1,16,0)  OutScaling=[]
  wires:
  Constant/1 -> Mux1/1
  Constant1/1 -> Mux1/2
  Subsystem/1("LL, deg") -> Mux1/3
  Subsystem/2("A, m") -> Mux1/4
  XYZ_LTP/1 -> Subsystem/1("XYZ, ltp"), Selector/1, Selector1/1, Selector3/1, Selector6/1
  Vx,y,z[NED]/1 -> Reshape/1  "cmd IAS"
  Mux1/1 -> Sensors/1
  Acc,x,y,z/1 -> Reshape1/1
  p,q,r/1 -> Mux1/7
  Constant3/1 -> Mux1/10
  Constant2/1 -> Mux1/11
  ISA Atmosphere Model/4(Air Density (Kg/m^3)) -> Dynamic Pressure/2, Mux3/6  "density"
  ISA Atmosphere Model/1(Temperature (K)) -> Mux1/9
  Mux2/1 -> Mux1/8
  ISA Atmosphere Model/3("Air Pressure (N/m^2) ") -> Mux2/1  "Pstat"
  ISA Atmosphere Model/2("Speed of Sound (m/s) ") -> Terminator4/1
  Dynamic Pressure/1 -> Mux2/2  "Pdyn"
  Selector/1 -> ISA Atmosphere Model/1(height (m))
  Reshape/1 -> Mux1/5, Reshape2/1, norm/1(In1)
  Reshape1/1 -> Mux1/6
  Reshape2/1 -> Dynamic Pressure/1
  Href/1 -> Subsystem/2(Href)
  Mux3/1 -> Estimates/1
  Constant4/1 -> Mux3/1
  Constant5/1 -> Mux3/2  "Wind North/East"
  Constant6/1 -> Mux3/3
  Attitude/1 -> Selector2/1, Selector5/1, Mux3/4
  Selector1/1 -> Mux3/5  "Baro altitude"
  norm/1(Out1) -> Mux3/7  "TAS"
  Constant7/1 -> Mux3/8
  Mux4/1 -> States/1
  Constant8/1 -> Mux4/1  "Reserved (not used)"
  Constant9/1 -> Mux4/2  "Global ON"
  Constant10/1 -> Mux4/6  "Slope_ON (not used)"
  Attitude_dot/1 -> Selector4/1
  Constant11/1 -> Mux4/9  "Yaw_ON (Rud)"
  Mux5/1 -> Commands/1
  Constant18/1 -> Mux5/1  "CmdPdynShift"
  ISA Atmosphere Model1/1(Temperature (K)) -> Terminator1/1
  ISA Atmosphere Model1/2("Speed of Sound (m/s) ") -> Terminator2/1
  ISA Atmosphere Model1/3("Air Pressure (N/m^2) ") -> Terminator3/1
  ISA Atmosphere Model1/4(Air Density (Kg/m^3)) -> Dynamic Pressure4/2
  Dynamic Pressure4/1 -> Mux5/2
  Mux9/1 -> Dynamic Pressure4/1  "cmd IAS"
  [Alt_ref] -> ISA Atmosphere Model1/1(height (m)), Mux5/7  "cmd altitude"
  [PitchAngle_ref] -> Mux5/3  "CmdPitchAngle"
  Constant22/1 -> Mux5/4  "CmdSlopeAngle"
  Constant24/1 -> Mux5/6  "CmdTouchDownLon"
  Constant23/1 -> Mux5/5  "CmdTouchDownLat"
  Constant25/1 -> Mux5/8  "CmdFlap"
  Constant26/1 -> Mux5/9  "CmdTurnRateShift"
  [TurnRate_ref] -> Mux5/10  "CmdTurnRate"
  Constant28/1 -> Mux5/11  "waypoint1"
  Constant29/1 -> Mux5/12  "waypoint2"
  Constant30/1 -> Mux5/13  "(OrbRadius OrbSense)"
  Mux6/1 -> Limits/1
  Constant31/1 -> Mux6/1  "LimReserved0"
  Constant33/1 -> Mux6/21  "LimReserved2"
  Constant32/1 -> Mux6/20  "LimReserved1"
  ISA Atmosphere Model2/1(Temperature (K)) -> Terminator5/1
  ISA Atmosphere Model2/2("Speed of Sound (m/s) ") -> Terminator6/1
  ISA Atmosphere Model2/3("Air Pressure (N/m^2) ") -> Terminator7/1
  ISA Atmosphere Model2/4(Air Density (Kg/m^3)) -> Dynamic Pressure2/2, Dynamic Pressure3/2
  Constant13/1 -> Dynamic Pressure2/1
  Constant34/1 -> Dynamic Pressure3/1
  Selector6/1 -> ISA Atmosphere Model2/1(height (m))
  Dynamic Pressure2/1 -> Mux6/2  "LimPdynMin"
  Dynamic Pressure3/1 -> Mux6/3  "LimPdynMax"
  Constant36/1 -> Mux6/4  "LimSlopeMin"
  Constant37/1 -> Mux6/5  "LimSlopeMax"
  Constant38/1 -> Mux6/6  "LimAltMin"
  Constant39/1 -> Mux6/7  "LimAltMax"
  Constant40/1 -> Mux6/8  "LimBankMin"
  Constant41/1 -> Mux6/9  "LimBankMax"
  Constant42/1 -> Mux6/10  "LimAileronMin"
  Constant43/1 -> Mux6/11  "LimAileronMax"
  Constant44/1 -> Mux6/12  "LimElevatorMin"
  Constant45/1 -> Mux6/13  "LimElevatorMax"
  Constant46/1 -> Mux6/14  "LimRudderMin"
  Constant47/1 -> Mux6/15  "LimRdderMax"
  Constant48/1 -> Mux6/16  "LimThrottleMin"
  Constant49/1 -> Mux6/17  "LimThrottleMax"
  Constant50/1 -> Mux6/18  "LimFlapsMin"
  Constant51/1 -> Mux6/19  "LimFlapsMax"
  Mux7/1 -> Gains/1
  Constant52/1 -> Mux7/1  "Reserved0"
  Constant53/1 -> Mux7/2  "PdynPID"
  Constant54/1 -> Mux7/3  "PitchAnglePID"
  Constant55/1 -> Mux7/4  "AltPID"
  Constant58/1 -> Mux7/6  "TurnRateHoldPID"
  Constant57/1 -> Mux7/5  "SlopeConv"
  Constant56/1 -> Mux7/7  "RollPID"
  Constant59/1 -> Mux7/8  "YawPID"
  Constant60/1 -> Mux7/9  "TrackPID"
  Constant61/1 -> Mux7/10  "TrackConv"
  Constant62/1 -> Mux7/11  "SlopeElevator (Alt)"
  Constant63/1 -> Mux7/12  "Reserved3"
  Mux8/1 -> Settings/1
  Constant64/1 -> Mux8/1  "Reserved0"
  Constant65/1 -> Mux8/2  "PSL"
  Constant66/1 -> Mux8/3  "Reserved1"
  Constant67/1 -> Mux8/5  "Reserved2"
  Constant68/1 -> Mux8/7  "Reserved3"
  Constant69/1 -> Mux8/9  "Reserved4"
  Constant70/1 -> Mux8/10  "ThrottleTrim"
  Constant71/1 -> Mux8/11  "LandingFlap"
  Constant72/1 -> Mux8/12  "Reserved6"
  Constant73/1 -> Mux8/4  "AileronTrim"
  Constant74/1 -> Mux8/6  "ElevatorTrim"
  Constant75/1 -> Mux8/8  "RudderTrim"
  Constant76/1 -> Mux4/7  "TurnRate_ON (Ail)"
  Constant77/1 -> Mux4/8  "Roll_ON (Ail)"
  Constant78/1 -> Mux4/4  "Pitch_ON"
  Constant79/1 -> Mux4/3  "Pdyn_ON"
  Constant80/1 -> Mux4/5  "Alt_ON"
  Constant81/1 -> Mux4/10  "TurnComp_ON (Elev)"
  Constant12/1 -> Mux4/11  "Alt2Elev_ON"
  Constant19/1 -> Mux4/12  "Tracker_ON"
  Constant14/1 -> Mux4/13  "AltToPdyn_ON"
  Constant15/1 -> Mux4/14  "Flap_ON"
  Constant16/1 -> Mux4/15  "Mode::Flying"
  Constant17/1 -> Mux4/16  "Manual::Standart"
  References/1 -> Demux/1
  Demux/1 -> [IAS_ref]
  Demux/2 -> [Alt_ref]
  Demux/3 -> [PitchAngle_ref]
  Demux/4 -> [TurnRate_ref]
  Constant20/1 -> Mux9/2
  [IAS_ref] -> Mux9/1

== system HILModelFull/Plant Model/Generic Sensor ==
  Sens : Inport
  Dynamics : Subsystem
  Measurement bias : Constant  Value=g_bias
  Product : Product  Multiplication=Matrix(*)  SaturateOnIntegerOverflow=on
  Random bias : simulink/Sources/Band-Limited White Noise  SystemSampleTime=-1  Cov=g_pow  Ts=g_Ts  seed=g_seeds(1:3)
  Saturation : Saturate  UpperLimit=g_sat(4:6)  LowerLimit=g_sat(1:3)
  "Scale factors & Cross-coupling  errors " : Constant  Value=g_sf_cc
  Sum1 : Sum  Inputs=|++  SaturateOnIntegerOverflow=on
  Sum4 : Sum  Inputs=++|  SaturateOnIntegerOverflow=on
  Zero-Order Hold : ZeroOrderHold  SampleTime=g_Ts
  Meas : Outport
  wires:
  Zero-Order Hold/1 -> Product/2
  Dynamics/1(Sens Dyn) -> Sum1/1
  Sum1/1 -> Saturation/1
  Sens/1 -> Zero-Order Hold/1
  Saturation/1 -> Meas/1
  Random bias/1 -> Sum1/2
  "Scale factors & Cross-coupling  errors "/1 -> Product/1
  Sum4/1 -> Dynamics/1("Sens ")
  Product/1 -> Sum4/1
  Measurement bias/1 -> Sum4/2

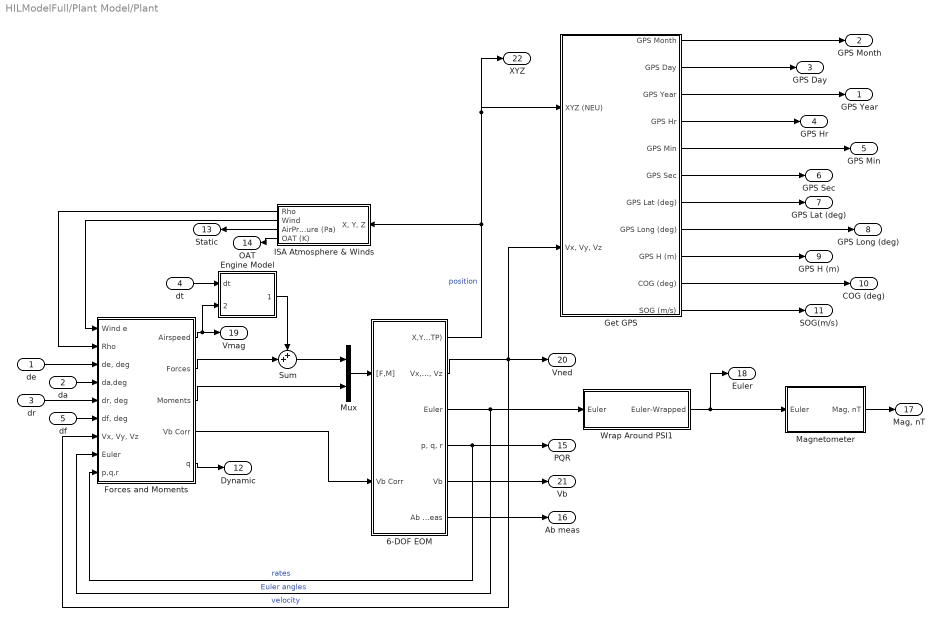
== system HILModelFull/Plant Model/Plant ==
  de : Inport
  da : Inport  Port=2
  dr : Inport  Port=3
  dt : Inport  Port=4
  df : Inport  Port=5
  6-DOF EOM : Subsystem
  Engine Model : Subsystem
  Forces and Moments : Subsystem
  Get GPS : Subsystem
  ISA Atmosphere & Winds : Subsystem  Orientation=left
  Magnetometer : Subsystem  mask{magField=[ 23143.6 5858.2 45511.9]}
      mask prompts: magField "Local Magnetic Field"
      mask help:
      | Simulates the Data from magnetometers with no noise.
      |
      | You can obtain data for the local magnetic field at:
      |
      | http://www.ngdc.noaa.gov/geomagmodels/IGRFWMM.jsp
  Mux : Mux  Inputs=2
  Sum : Sum  Inputs=++|  SaturateOnIntegerOverflow=on
  Wrap Around PSI1 : Subsystem
  GPS Year : Outport
  GPS Month : Outport  Port=2
  GPS Day : Outport  Port=3
  GPS Hr : Outport  Port=4
  GPS Min : Outport  Port=5
  GPS Sec : Outport  Port=6
  GPS Lat (deg) : Outport  Port=7
  GPS Long (deg) : Outport  Port=8
  GPS H (m) : Outport  Port=9
  COG (deg) : Outport  Port=10
  SOG(m/s) : Outport  Port=11
  Dynamic : Outport  Port=12
  Static : Outport  Orientation=left  Port=13
  OAT : Outport  Orientation=left  Port=14
  PQR : Outport  Port=15
  Ab meas : Outport  Port=16
  "Mag, nT" : Outport  Port=17
  Euler : Outport  Port=18
  Vmag : Outport  Port=19
  Vned : Outport  Port=20
  Vb : Outport  Port=21
  XYZ : Outport  Port=22
  wires:
  Get GPS/1(GPS Month) -> GPS Month/1
  Get GPS/2(GPS Day) -> GPS Day/1
  Get GPS/3(GPS Year) -> GPS Year/1
  Get GPS/4(GPS Hr) -> GPS Hr/1
  Get GPS/5(GPS Min) -> GPS Min/1
  Get GPS/6(GPS Sec) -> GPS Sec/1
  Get GPS/7(GPS Lat (deg)) -> GPS Lat (deg)/1
  Get GPS/8(GPS Long (deg)) -> GPS Long (deg)/1
  Get GPS/9(GPS H (m)) -> GPS H (m)/1
  6-DOF EOM/6(Ab meas) -> Ab meas/1
  Mux/1 -> 6-DOF EOM/1("[F,M]")
  6-DOF EOM/5(Vb) -> Vb/1
  Engine Model/1(Thrust) -> Sum/1
  Forces and Moments/5(q) -> Dynamic/1
  ISA Atmosphere & Winds/3(AirPressure (Pa)) -> Static/1
  Forces and Moments/1(Airspeed) -> Engine Model/2(Vmag), Vmag/1
  ISA Atmosphere & Winds/2(Wind) -> Forces and Moments/1(Wind e)
  ISA Atmosphere & Winds/1(Rho) -> Forces and Moments/2(Rho)
  Forces and Moments/3(Moments) -> Mux/2
  Forces and Moments/2(Forces) -> Sum/2
  Sum/1 -> Mux/1
  Forces and Moments/4(Vb Corr) -> 6-DOF EOM/2(Vb Corr)
  6-DOF EOM/1(X,Y,Z (LTP)) -> ISA Atmosphere & Winds/1("X, Y, Z"), Get GPS/1(XYZ (NEU)), XYZ/1  "position"
  6-DOF EOM/2("Vx, Vy, Vz") -> Vned/1, Forces and Moments/7("Vx, Vy, Vz "), Get GPS/2("Vx, Vy, Vz")  "velocity"
  6-DOF EOM/3(Euler) -> Forces and Moments/8(Euler), Wrap Around PSI1/1(Euler)  "Euler angles"
  6-DOF EOM/4("p, q, r") -> PQR/1, Forces and Moments/9(p,q,r)  "rates"
  dt/1 -> Engine Model/1(dt)
  de/1 -> Forces and Moments/3("de, deg")
  da/1 -> Forces and Moments/4(da,deg)
  dr/1 -> Forces and Moments/5("dr, deg")
  df/1 -> Forces and Moments/6("df, deg")
  Wrap Around PSI1/1(Euler-Wrapped) -> Euler/1, Magnetometer/1(Euler)
  Magnetometer/1("Mag, nT") -> "Mag, nT"/1
  Get GPS/10(COG (deg)) -> COG (deg)/1
  Get GPS/11(SOG (m/s)) -> SOG(m/s)/1
  ISA Atmosphere & Winds/4(OAT (K)) -> OAT/1

== system HILModelFull/Plant Model/Subsystem ==
  PQR : Inport
  Ab : Inport  Port=2
  Mag : Inport  Port=3
  Mux2 : Mux  Inputs=3
  Three-axis Accelerometer : aerolibnav/Three-axis Accelerometer  SystemSampleTime=-1  units=Metric (MKS)  acc=[0 0 0]  gtype=off  dtype_a=on  w_a=190  z_a=0.707  a_sf_cc=[-41 0 0; 0 41 0; 0 0 -43]  a_bias=[2015 2018 2006]  a_rand=off  a_seeds=[23093 23094 23095]  a_pow=[0.008 0.008 0.008]  a_sat="[-inf  -inf  -inf  inf inf inf]"  a_Ts=SampleT
  Three-axis Gyroscope : aerolibnav/Three-axis Gyroscope  SystemSampleTime=-1  dtype_g=off  w_g=190  z_g=0.707  g_sf_cc=[-142 0 0; 0 142 0; 0 0 235]  g_bias=[1866 1981 2042]  g_sen=[0 0 0]  g_rand=off  g_seeds=[23093 23094 23095]  g_pow=[0.008 0.008 0.008]  g_sat="[-inf  -inf  -inf  inf inf inf]"  g_Ts=SampleT
  Sens : Outport
  wires:
  Three-axis Gyroscope/1 -> Mux2/1
  Three-axis Accelerometer/1 -> Mux2/2
  PQR/1 -> Three-axis Gyroscope/1
  Ab/1 -> Three-axis Accelerometer/1
  Mux2/1 -> Sens/1
  Mag/1 -> Mux2/3
